simulink model "model2"  (Simulink 7.7)
settings: Solver=ode45  StartTime=0.0  StopTime=10.0  RelTol=1e-3
values from neighbouring files (symbols this model uses):
  lim = limit((gamma(n) / (gamma(n * 3 - 1))) / (gamma(n - 1) / (3 * gamma(n - 1))), n, inf)    [dalamber_condition.m]    (also in koshi_condition.m = limit((((n + 1) / (2 * n - 3))^(n^2)) ^ (1 / n), n, inf); leibnic_condition.m = limit(cos(n) / (n ^ 2), n, inf); nessary_condition.m = limit((n + 1) / (2 * n + 1), n, inf); uslovn_absolut.m = limit((log(2 * n / (n + 2)) ^ n) ^ (1 / n), n, inf))
libraries: simulink x3
settings Model: Creator=ozisoft  LastModifiedBy=ozisoft

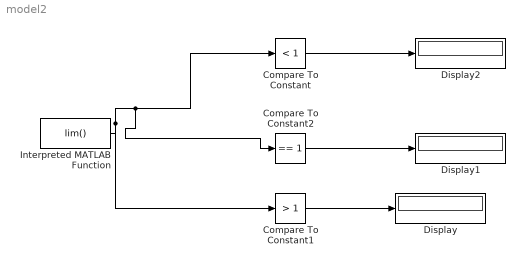
== system model2 ==
  Compare To Constant : simulink/Logic and Bit Operations/Compare To Constant  SystemSampleTime=-1  relop=<  const=1  LogicOutDataTypeMode=uint8
  Compare To Constant1 : simulink/Logic and Bit Operations/Compare To Constant  SystemSampleTime=-1  relop=>  const=1  LogicOutDataTypeMode=uint8
  Compare To Constant2 : simulink/Logic and Bit Operations/Compare To Constant  SystemSampleTime=-1  relop===  const=1  LogicOutDataTypeMode=uint8
  Display : Display
  Display1 : Display
  Display2 : Display
  Interpreted MATLAB Function : MATLABFcn  MATLABFcn=lim()  OutputSignalType=real
  wires:
  Interpreted MATLAB Function/1 -> Compare To Constant/1, Compare To Constant2/1, Compare To Constant1/1
  Compare To Constant1/1 -> Display/1
  Compare To Constant2/1 -> Display1/1
  Compare To Constant/1 -> Display2/1
